simulink model "product_b1"  (R2021a)
settings: Solver=VariableStepAuto  StartTime=0.0  StopTime=10  FixedStep=0.001  RelTol=1e-3
InitFcn:
  | PreFunction.BusData
values from neighbouring files (symbols this model uses):
  N = 10    [TrajectoryGenerator.m]
undefined symbols (not defined in the file or in its folder): X, Y, Z
libraries: nesl_utility x29, sm_lib x24
settings Model: Creator=hanli  LastModifiedBy=hanli

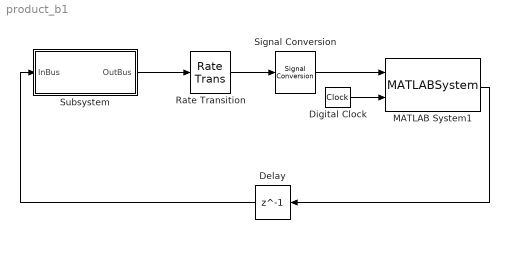
== system product_b1 ==
  Delay : Delay  DelayLength=1  InitialCondition=0  SampleTime=0.001
  Digital Clock : DigitalClock
  MATLAB System1 : MATLABSystem  System=EmptyController  SimulateUsing=Code generation
      mask Type: EmptyController
      mask Display:
      | disp('EmptyController');
      | port_label('input',1,'u');
      | port_label('input',2,'t');
      | port_label('output',1,'y');
  Rate Transition : RateTransition  OutPortSampleTime=0.001
  Signal Conversion : SignalConversion  ConversionOutput=Nonvirtual bus  OutDataTypeStr=Bus: AmberB1OutBus  OverrideOpt=off
  Subsystem : Subsystem
  wires:
  Subsystem/1(OutBus) -> Rate Transition/1
  Rate Transition/1 -> Signal Conversion/1
  Signal Conversion/1 -> MATLAB System1/1
  Delay/1 -> Subsystem/1(InBus)
  MATLAB System1/1 -> Delay/1
  Digital Clock/1 -> MATLAB System1/2

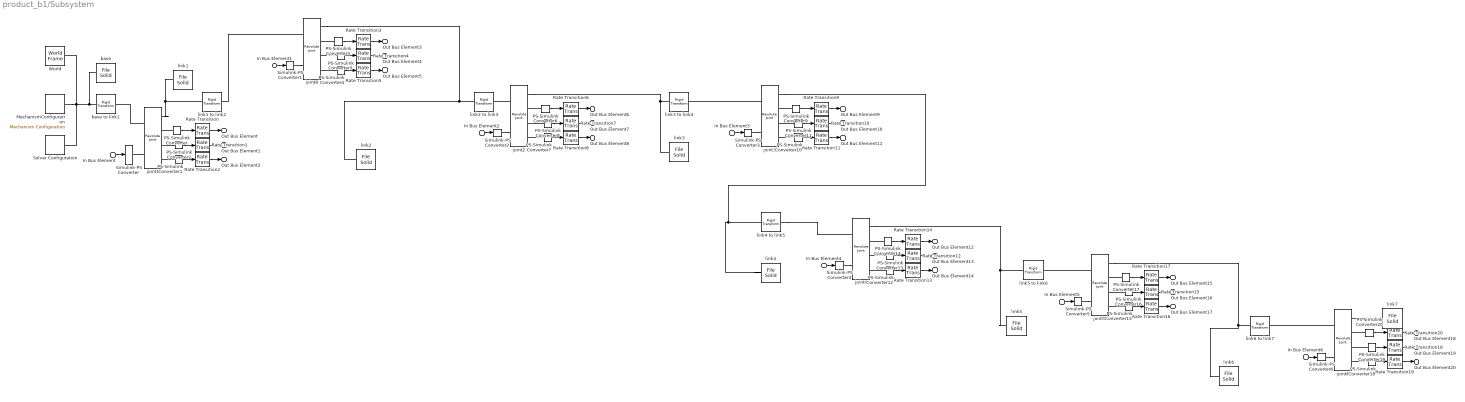
== system product_b1/Subsystem ==
  In Bus Element : Inport  PortName=InBus  Element=position_1
  In Bus Element1 : Inport  PortName=InBus  Element=position_2
  In Bus Element2 : Inport  PortName=InBus  Element=position_3
  In Bus Element3 : Inport  PortName=InBus  Element=position_4
  In Bus Element4 : Inport  PortName=InBus  Element=position_5
  In Bus Element5 : Inport  PortName=InBus  Element=position_6
  In Bus Element6 : Inport  PortName=InBus  Element=position_7
  MechanismConfiguration : sm_lib/Utilities/Mechanism Configuration  UniformGravity=Constant  GravityVector=[0 0 -9.80665]  GravityVectorUnits=m/s^2  GravityUnits=m/s^2  LinearizationDelta=0.001  JointModeTransitionNonlinearIterations=2
  PS-Simulink Converter{,1..20} (21 alike) : nesl_utility/PS-Simulink Converter  PhysicalDomain=network_engine_domain  SubClassName=ps_output  LeftPortType=input  RightPortType=output  PseudoPeriodic=off  Frequencies=[]  Unit=inherit  AffineConversion=off
      settings: SourceProductBaseCode=PW,SS
  Rate Transition{,1..20} (21 alike) : RateTransition  OutPortSampleTime=0.001
  Simulink-PS Converter{,1..6} (7 alike) : nesl_utility/Simulink-PS Converter  PhysicalDomain=network_engine_domain  SubClassName=ps_input  LeftPortType=input  RightPortType=output  PseudoPeriodic=off  Frequencies=[]  NoiseDistribution=none  NoiseParameters=[]  Unit=rad  AffineConversion=off  FilteringAndDerivatives=filter  SimscapeFilterOrder=2  InputFilterTimeConstant=0.001  UdotUserProvided=0
      settings: SourceProductBaseCode=PW,SS
  Solver Configuration : nesl_utility/Solver Configuration  PhysicalDomain=network_engine_domain  SubClassName=solver  LeftPortType=input  RightPortType=generic  Tones=[]  Harmonics=[]  SimulateNoise=off  Profile=off  UseLocalSampling=off  EnableSwitchedLinearOptims=on  FrequencyDomain=off  UseCCode=off  RelTol=0.001  AbsTol=1e-06  MinStep=1e-09  ToWorkspace=off  RevertToSquareIcSolve=off  NumHomotopyIterations=100  PhasorMode=off  PhasorModeNumHarmonics=1  DoDC=off  ResidualTolerance=1e-09  UseLocalSolver=off  LocalSolverChoice=NE_BACKWARD_EULER_ADVANCER  LocalSolverSampleTime=0.001  DoFixedCost=off  MaxNonlinIter=3  MaxModeIter=2  ComputeImpulses=off  ImpulseIterations=2  LinearAlgebra=auto  EquationFormulation=NE_TIME_EF  DelaysMemoryBudget=1024  AutomaticFiltering=on  FilteringTimeConstant=0.001  PartitionStorageMethod=AS_NEEDED  PartitionMemoryBudget=1024  PartitionMethod=ROBUST
      settings: SourceProductBaseCode=PW,SS
  World : sm_lib/Frames and Transforms/World Frame
  base : sm_lib/Body Elements/File Solid  ExtGeomFileName=meshes/base_link.STL  UnitType=Custom  ExtGeomFileUnits=m  StepReaderType=HEX  ExportConvexHullGeometry=off  InertiaType=Custom  Mass=0.26734  MassUnits=kg  CenterOfMass=[6.237e-05, 0.00031998, 0.048235]  CenterOfMassUnits=m  MomentsOfInertia=[0.00029777, 0.00024467, 0.00035934]  MomentsOfInertiaUnits=kg*m^2  ProductsOfInertia=[2.2995e-07, -3.3641e-08, 5.8953e-08]  ProductsOfInertiaUnits=kg*m^2  BasedOnType=DensityFromFile  Density=1000  DensityUnits=kg/m^3  DoExposeReferenceFrame=on  SerializedFrames=<Frames/>  GraphicType=FromGeometry  MarkerShape=Sphere  MarkerSize=10  GraphicVisPropType=SimpleVisualProperties  GraphicDiffuseColor=[0.62745, 0.62745, 0.62745]  GraphicSpecularColor=[0.5 0.5 0.5 1.0]  GraphicAmbientColor=[0.15 0.15 0.15 1.0]  GraphicEmissiveColor=[0.0 0.0 0.0 1.0]  GraphicShininess=75  GraphicOpacity=1
  base to link1 : sm_lib/Frames and Transforms/Rigid Transform  TranslationMethod=Cartesian  TranslationStandardOffset=0  TranslationLengthUnit=m  TranslationStandardAxis=+Z  TranslationCartesianOffset=[0, 0, 0.082]  TranslationROffset=0  TranslationROffsetUnits=m  TranslationZOffset=0  TranslationZOffsetUnits=m  TranslationThetaOffset=0  TranslationThetaOffsetUnits=deg  RotationMethod=RotationSequence  RotationAngleUnits=deg  RotationStandardAxis=+Z  RotationAngle=0.0  RotationArbitraryAxis=[0 0 1]  FollAlignAxisA=+X  BaseAlignAxisA=+Y  FollAlignAxisB=+Y  BaseAlignAxisB=+Z  RotationSequenceAxes=BaseAxes  RotationSequence=XYZ  RotationSequenceAngles=[0, 0, 0]  RotationSequenceAnglesUnits=rad  RotationMatrix=[1 0 0; 0 1 0; 0 0 1]
  joint1 : sm_lib/Joints/Revolute Joint  JointMode=Normal  SenseConstraintForce=off  SenseConstraintForceX=off  SenseConstraintForceY=off  SenseConstraintForceZ=off  SenseConstraintTorque=off  SenseConstraintTorqueX=off  SenseConstraintTorqueY=off  SenseConstraintTorqueZ=off  SenseTotalForce=off  SenseTotalForceX=off  SenseTotalForceY=off  SenseTotalForceZ=off  SenseTotalTorque=off  SenseTotalTorqueX=off  SenseTotalTorqueY=off  SenseTotalTorqueZ=off  CompositeWrenchDir=FollowerOnBase  CompositeWrenchFrame=BaseFrame  EquilibriumPosition=0  EquilibriumPositionUnits=deg  SpringStiffness=0  SpringStiffnessUnits=N*m/deg  DampingCoefficient=0.1  DampingCoefficientUnits=m^2*kg/s/rad  TorqueActuationMode=ComputedTorque  MotionActuationMode=InputMotion  SensePosition=on  SenseVelocity=on  SenseAcceleration=off  SenseTorqueForce=on  SenseLowerLimitTorqueForce=off  SenseUpperLimitTorqueForce=off  LowerLimitSpecify=on  LowerLimitBound=-2.4435  LowerLimitBoundUnits=rad  LowerLimitStiffness=1e4  LowerLimitStiffnessUnits=N*m/deg  LowerLimitDamping=10  LowerLimitDampingUnits=N*m/(deg/s)  LowerLimitTransitionRegionWidth=0.1  LowerLimitTransitionRegionWidthUnits=deg  UpperLimitSpecify=on  UpperLimitBound=2.4435  UpperLimitBoundUnits=rad  UpperLimitStiffness=1e4  UpperLimitStiffnessUnits=N*m/deg  UpperLimitDamping=10  UpperLimitDampingUnits=N*m/(deg/s)  UpperLimitTransitionRegionWidth=0.1  UpperLimitTransitionRegionWidthUnits=deg  PositionTargetSpecify=off  PositionTargetPriority=High  PositionTargetValue=0  PositionTargetValueUnits=deg  VelocityTargetSpecify=off  VelocityTargetPriority=High  VelocityTargetValue=0  VelocityTargetValueUnits=deg/s
  joint{2..5} (4 alike) : sm_lib/Joints/Revolute Joint  JointMode=Normal  SenseConstraintForce=off  SenseConstraintForceX=off  SenseConstraintForceY=off  SenseConstraintForceZ=off  SenseConstraintTorque=off  SenseConstraintTorqueX=off  SenseConstraintTorqueY=off  SenseConstraintTorqueZ=off  SenseTotalForce=off  SenseTotalForceX=off  SenseTotalForceY=off  SenseTotalForceZ=off  SenseTotalTorque=off  SenseTotalTorqueX=off  SenseTotalTorqueY=off  SenseTotalTorqueZ=off  CompositeWrenchDir=FollowerOnBase  CompositeWrenchFrame=BaseFrame  EquilibriumPosition=0  EquilibriumPositionUnits=deg  SpringStiffness=0  SpringStiffnessUnits=N*m/deg  DampingCoefficient=0.1  DampingCoefficientUnits=m^2*kg/s/rad  TorqueActuationMode=ComputedTorque  MotionActuationMode=InputMotion  SensePosition=on  SenseVelocity=on  SenseAcceleration=off  SenseTorqueForce=on  SenseLowerLimitTorqueForce=off  SenseUpperLimitTorqueForce=off  LowerLimitSpecify=on  LowerLimitBound=-2.2863  LowerLimitBoundUnits=rad  LowerLimitStiffness=1e4  LowerLimitStiffnessUnits=N*m/deg  LowerLimitDamping=10  LowerLimitDampingUnits=N*m/(deg/s)  LowerLimitTransitionRegionWidth=0.1  LowerLimitTransitionRegionWidthUnits=deg  UpperLimitSpecify=on  UpperLimitBound=2.2863  UpperLimitBoundUnits=rad  UpperLimitStiffness=1e4  UpperLimitStiffnessUnits=N*m/deg  UpperLimitDamping=10  UpperLimitDampingUnits=N*m/(deg/s)  UpperLimitTransitionRegionWidth=0.1  UpperLimitTransitionRegionWidthUnits=deg  PositionTargetSpecify=off  PositionTargetPriority=High  PositionTargetValue=0  PositionTargetValueUnits=deg  VelocityTargetSpecify=off  VelocityTargetPriority=High  VelocityTargetValue=0  VelocityTargetValueUnits=deg/s
  joint6 : sm_lib/Joints/Revolute Joint  JointMode=Normal  SenseConstraintForce=off  SenseConstraintForceX=off  SenseConstraintForceY=off  SenseConstraintForceZ=off  SenseConstraintTorque=off  SenseConstraintTorqueX=off  SenseConstraintTorqueY=off  SenseConstraintTorqueZ=off  SenseTotalForce=off  SenseTotalForceX=off  SenseTotalForceY=off  SenseTotalForceZ=off  SenseTotalTorque=off  SenseTotalTorqueX=off  SenseTotalTorqueY=off  SenseTotalTorqueZ=off  CompositeWrenchDir=FollowerOnBase  CompositeWrenchFrame=BaseFrame  EquilibriumPosition=0  EquilibriumPositionUnits=deg  SpringStiffness=0  SpringStiffnessUnits=N*m/deg  DampingCoefficient=0.1  DampingCoefficientUnits=m^2*kg/s/rad  TorqueActuationMode=ComputedTorque  MotionActuationMode=InputMotion  SensePosition=on  SenseVelocity=on  SenseAcceleration=off  SenseTorqueForce=on  SenseLowerLimitTorqueForce=off  SenseUpperLimitTorqueForce=off  LowerLimitSpecify=off  LowerLimitBound=-2.2863  LowerLimitBoundUnits=rad  LowerLimitStiffness=1e4  LowerLimitStiffnessUnits=N*m/deg  LowerLimitDamping=10  LowerLimitDampingUnits=N*m/(deg/s)  LowerLimitTransitionRegionWidth=0.1  LowerLimitTransitionRegionWidthUnits=deg  UpperLimitSpecify=off  UpperLimitBound=2.2863  UpperLimitBoundUnits=rad  UpperLimitStiffness=1e4  UpperLimitStiffnessUnits=N*m/deg  UpperLimitDamping=10  UpperLimitDampingUnits=N*m/(deg/s)  UpperLimitTransitionRegionWidth=0.1  UpperLimitTransitionRegionWidthUnits=deg  PositionTargetSpecify=off  PositionTargetPriority=High  PositionTargetValue=0  PositionTargetValueUnits=deg  VelocityTargetSpecify=off  VelocityTargetPriority=High  VelocityTargetValue=0  VelocityTargetValueUnits=deg/s
  joint8 : sm_lib/Joints/Revolute Joint  JointMode=Normal  SenseConstraintForce=off  SenseConstraintForceX=off  SenseConstraintForceY=off  SenseConstraintForceZ=off  SenseConstraintTorque=off  SenseConstraintTorqueX=off  SenseConstraintTorqueY=off  SenseConstraintTorqueZ=off  SenseTotalForce=off  SenseTotalForceX=off  SenseTotalForceY=off  SenseTotalForceZ=off  SenseTotalTorque=off  SenseTotalTorqueX=off  SenseTotalTorqueY=off  SenseTotalTorqueZ=off  CompositeWrenchDir=FollowerOnBase  CompositeWrenchFrame=BaseFrame  EquilibriumPosition=0  EquilibriumPositionUnits=deg  SpringStiffness=0  SpringStiffnessUnits=N*m/deg  DampingCoefficient=0.1  DampingCoefficientUnits=m^2*kg/s/rad  TorqueActuationMode=ComputedTorque  MotionActuationMode=InputMotion  SensePosition=on  SenseVelocity=on  SenseAcceleration=off  SenseTorqueForce=on  SenseLowerLimitTorqueForce=off  SenseUpperLimitTorqueForce=off  LowerLimitSpecify=on  LowerLimitBound=-2.3213  LowerLimitBoundUnits=rad  LowerLimitStiffness=1e4  LowerLimitStiffnessUnits=N*m/deg  LowerLimitDamping=10  LowerLimitDampingUnits=N*m/(deg/s)  LowerLimitTransitionRegionWidth=0.1  LowerLimitTransitionRegionWidthUnits=deg  UpperLimitSpecify=on  UpperLimitBound=2.3213  UpperLimitBoundUnits=rad  UpperLimitStiffness=1e4  UpperLimitStiffnessUnits=N*m/deg  UpperLimitDamping=10  UpperLimitDampingUnits=N*m/(deg/s)  UpperLimitTransitionRegionWidth=0.1  UpperLimitTransitionRegionWidthUnits=deg  PositionTargetSpecify=off  PositionTargetPriority=High  PositionTargetValue=0  PositionTargetValueUnits=deg  VelocityTargetSpecify=off  VelocityTargetPriority=High  VelocityTargetValue=0  VelocityTargetValueUnits=deg/s
  link1 : sm_lib/Body Elements/File Solid  ExtGeomFileName=meshes/link1.STL  UnitType=Custom  ExtGeomFileUnits=m  StepReaderType=HEX  ExportConvexHullGeometry=off  InertiaType=Custom  Mass=0.2539  MassUnits=kg  CenterOfMass=[-7.1956e-05, -0.0006525, 0.065648]  CenterOfMassUnits=m  MomentsOfInertia=[0.00013206, 0.00021227, 0.00013113]  MomentsOfInertiaUnits=kg*m^2  ProductsOfInertia=[-7.2775e-06, 5.8071e-08, -1.112e-07]  ProductsOfInertiaUnits=kg*m^2  BasedOnType=DensityFromFile  Density=1000  DensityUnits=kg/m^3  DoExposeReferenceFrame=on  SerializedFrames=<Frames/>  GraphicType=FromGeometry  MarkerShape=Sphere  MarkerSize=10  GraphicVisPropType=SimpleVisualProperties  GraphicDiffuseColor=[0.83922, 0.44706, 0.38431]  GraphicSpecularColor=[0.5 0.5 0.5 1.0]  GraphicAmbientColor=[0.15 0.15 0.15 1.0]  GraphicEmissiveColor=[0.0 0.0 0.0 1.0]  GraphicShininess=75  GraphicOpacity=1
  link1 to link2 : sm_lib/Frames and Transforms/Rigid Transform  TranslationMethod=Cartesian  TranslationStandardOffset=0  TranslationLengthUnit=m  TranslationStandardAxis=+Z  TranslationCartesianOffset=[0, 0.025, 0.08649999999999999]  TranslationROffset=0  TranslationROffsetUnits=m  TranslationZOffset=0  TranslationZOffsetUnits=m  TranslationThetaOffset=0  TranslationThetaOffsetUnits=deg  RotationMethod=RotationSequence  RotationAngleUnits=deg  RotationStandardAxis=+Z  RotationAngle=0.0  RotationArbitraryAxis=[0 0 1]  FollAlignAxisA=+X  BaseAlignAxisA=+Y  FollAlignAxisB=+Y  BaseAlignAxisB=+Z  RotationSequenceAxes=BaseAxes  RotationSequence=XYZ  RotationSequenceAngles=[1.5708, 0, 3.1416]  RotationSequenceAnglesUnits=rad  RotationMatrix=[1 0 0; 0 1 0; 0 0 1]
  link2 : sm_lib/Body Elements/File Solid  ExtGeomFileName=meshes/link2.STL  UnitType=Custom  ExtGeomFileUnits=m  StepReaderType=HEX  ExportConvexHullGeometry=off  InertiaType=Custom  Mass=0.26004  MassUnits=kg  CenterOfMass=[5.7141e-05, 0.080805, -0.0071326]  CenterOfMassUnits=m  MomentsOfInertia=[0.00027467, 0.00015654, 0.00029313]  MomentsOfInertiaUnits=kg*m^2  ProductsOfInertia=[-3.0164e-06, 9.7156e-08, 1.0052e-07]  ProductsOfInertiaUnits=kg*m^2  BasedOnType=DensityFromFile  Density=1000  DensityUnits=kg/m^3  DoExposeReferenceFrame=on  SerializedFrames=<Frames/>  GraphicType=FromGeometry  MarkerShape=Sphere  MarkerSize=10  GraphicVisPropType=SimpleVisualProperties  GraphicDiffuseColor=[0.66667, 0.66667, 0.66667]  GraphicSpecularColor=[0.5 0.5 0.5 1.0]  GraphicAmbientColor=[0.15 0.15 0.15 1.0]  GraphicEmissiveColor=[0.0 0.0 0.0 1.0]  GraphicShininess=75  GraphicOpacity=1
  link2 to link3 : sm_lib/Frames and Transforms/Rigid Transform  TranslationMethod=Cartesian  TranslationStandardOffset=0  TranslationLengthUnit=m  TranslationStandardAxis=+Z  TranslationCartesianOffset=[0, 0.1364, -0.025]  TranslationROffset=0  TranslationROffsetUnits=m  TranslationZOffset=0  TranslationZOffsetUnits=m  TranslationThetaOffset=0  TranslationThetaOffsetUnits=deg  RotationMethod=RotationSequence  RotationAngleUnits=deg  RotationStandardAxis=+Z  RotationAngle=0.0  RotationArbitraryAxis=[0 0 1]  FollAlignAxisA=+X  BaseAlignAxisA=+Y  FollAlignAxisB=+Y  BaseAlignAxisB=+Z  RotationSequenceAxes=BaseAxes  RotationSequence=XYZ  RotationSequenceAngles=[1.5708, 0, 3.1416]  RotationSequenceAnglesUnits=rad  RotationMatrix=[1 0 0; 0 1 0; 0 0 1]
  link3 : sm_lib/Body Elements/File Solid  ExtGeomFileName=meshes/link3.STL  UnitType=Custom  ExtGeomFileUnits=m  StepReaderType=HEX  ExportConvexHullGeometry=off  InertiaType=Custom  Mass=0.19745  MassUnits=kg  CenterOfMass=[7.536e-05, 0.00081876, 0.06766999999999999]  CenterOfMassUnits=m  MomentsOfInertia=[8.8302e-05, 0.00014017, 8.488e-05]  MomentsOfInertiaUnits=kg*m^2  ProductsOfInertia=[5.8084e-06, -9.7553e-08, -1.0051e-07]  ProductsOfInertiaUnits=kg*m^2  BasedOnType=DensityFromFile  Density=1000  DensityUnits=kg/m^3  DoExposeReferenceFrame=on  SerializedFrames=<Frames/>  GraphicType=FromGeometry  MarkerShape=Sphere  MarkerSize=10  GraphicVisPropType=SimpleVisualProperties  GraphicDiffuseColor=[0.83922, 0.44706, 0.38431]  GraphicSpecularColor=[0.5 0.5 0.5 1.0]  GraphicAmbientColor=[0.15 0.15 0.15 1.0]  GraphicEmissiveColor=[0.0 0.0 0.0 1.0]  GraphicShininess=75  GraphicOpacity=1
  link3 to link4 : sm_lib/Frames and Transforms/Rigid Transform  TranslationMethod=Cartesian  TranslationStandardOffset=0  TranslationLengthUnit=m  TranslationStandardAxis=+Z  TranslationCartesianOffset=[0, -0.025, 0.08110000000000001]  TranslationROffset=0  TranslationROffsetUnits=m  TranslationZOffset=0  TranslationZOffsetUnits=m  TranslationThetaOffset=0  TranslationThetaOffsetUnits=deg  RotationMethod=RotationSequence  RotationAngleUnits=deg  RotationStandardAxis=+Z  RotationAngle=0.0  RotationArbitraryAxis=[0 0 1]  FollAlignAxisA=+X  BaseAlignAxisA=+Y  FollAlignAxisB=+Y  BaseAlignAxisB=+Z  RotationSequenceAxes=BaseAxes  RotationSequence=XYZ  RotationSequenceAngles=[1.5708, 0, 0]  RotationSequenceAnglesUnits=rad  RotationMatrix=[1 0 0; 0 1 0; 0 0 1]
  link4 : sm_lib/Body Elements/File Solid  ExtGeomFileName=meshes/link4.STL  UnitType=Custom  ExtGeomFileUnits=m  StepReaderType=HEX  ExportConvexHullGeometry=off  InertiaType=Custom  Mass=0.2255  MassUnits=kg  CenterOfMass=[5.5658e-05, 0.075812, -0.010096]  CenterOfMassUnits=m  MomentsOfInertia=[0.00018432, 0.00014008, 0.00019346]  MomentsOfInertiaUnits=kg*m^2  ProductsOfInertia=[5.464e-09, 9.3583e-08, 9.341e-08]  ProductsOfInertiaUnits=kg*m^2  BasedOnType=DensityFromFile  Density=1000  DensityUnits=kg/m^3  DoExposeReferenceFrame=on  SerializedFrames=<Frames/>  GraphicType=FromGeometry  MarkerShape=Sphere  MarkerSize=10  GraphicVisPropType=SimpleVisualProperties  GraphicDiffuseColor=[0.66667, 0.66667, 0.66667]  GraphicSpecularColor=[0.5 0.5 0.5 1.0]  GraphicAmbientColor=[0.15 0.15 0.15 1.0]  GraphicEmissiveColor=[0.0 0.0 0.0 1.0]  GraphicShininess=75  GraphicOpacity=1
  link4 to link5 : sm_lib/Frames and Transforms/Rigid Transform  TranslationMethod=Cartesian  TranslationStandardOffset=0  TranslationLengthUnit=m  TranslationStandardAxis=+Z  TranslationCartesianOffset=[0, 0.121, -0.025]  TranslationROffset=0  TranslationROffsetUnits=m  TranslationZOffset=0  TranslationZOffsetUnits=m  TranslationThetaOffset=0  TranslationThetaOffsetUnits=deg  RotationMethod=RotationSequence  RotationAngleUnits=deg  RotationStandardAxis=+Z  RotationAngle=0.0  RotationArbitraryAxis=[0 0 1]  FollAlignAxisA=+X  BaseAlignAxisA=+Y  FollAlignAxisB=+Y  BaseAlignAxisB=+Z  RotationSequenceAxes=BaseAxes  RotationSequence=XYZ  RotationSequenceAngles=[-1.5708, 0, 0]  RotationSequenceAnglesUnits=rad  RotationMatrix=[1 0 0; 0 1 0; 0 0 1]
  link5 : sm_lib/Body Elements/File Solid  ExtGeomFileName=meshes/link5.STL  UnitType=Custom  ExtGeomFileUnits=m  StepReaderType=HEX  ExportConvexHullGeometry=off  InertiaType=Custom  Mass=0.188342091601826  MassUnits=kg  CenterOfMass=[-6.47608224975801e-05, -0.000135644729966451, 0.0681146474008698]  CenterOfMassUnits=m  MomentsOfInertia=[8.572084994320241e-05, 0.000135395618146542, 8.20376711496822e-05]  MomentsOfInertiaUnits=kg*m^2  ProductsOfInertia=[-5.79908404802222e-06, 9.3610025889588e-08, -9.362853198210679e-08]  ProductsOfInertiaUnits=kg*m^2  BasedOnType=DensityFromFile  Density=1000  DensityUnits=kg/m^3  DoExposeReferenceFrame=on  SerializedFrames=<Frames/>  GraphicType=FromGeometry  MarkerShape=Sphere  MarkerSize=10  GraphicVisPropType=SimpleVisualProperties  GraphicDiffuseColor=[0.83921568627451, 0.447058823529412, 0.384313725490196]  GraphicSpecularColor=[0.5 0.5 0.5 1.0]  GraphicAmbientColor=[0.15 0.15 0.15 1.0]  GraphicEmissiveColor=[0.0 0.0 0.0 1.0]  GraphicShininess=75  GraphicOpacity=1
  link5 to link6 : sm_lib/Frames and Transforms/Rigid Transform  TranslationMethod=Cartesian  TranslationStandardOffset=0  TranslationLengthUnit=m  TranslationStandardAxis=+Z  TranslationCartesianOffset=[0, 0.025, 0.08110000000000001]  TranslationROffset=0  TranslationROffsetUnits=m  TranslationZOffset=0  TranslationZOffsetUnits=m  TranslationThetaOffset=0  TranslationThetaOffsetUnits=deg  RotationMethod=RotationSequence  RotationAngleUnits=deg  RotationStandardAxis=+Z  RotationAngle=0.0  RotationArbitraryAxis=[0 0 1]  FollAlignAxisA=+X  BaseAlignAxisA=+Y  FollAlignAxisB=+Y  BaseAlignAxisB=+Z  RotationSequenceAxes=BaseAxes  RotationSequence=XYZ  RotationSequenceAngles=[-1.5708, 0, 0]  RotationSequenceAnglesUnits=rad  RotationMatrix=[1 0 0; 0 1 0; 0 0 1]
  link6 : sm_lib/Body Elements/File Solid  ExtGeomFileName=meshes/link6.STL  UnitType=Custom  ExtGeomFileUnits=m  StepReaderType=HEX  ExportConvexHullGeometry=off  InertiaType=Custom  Mass=0.228014101529845  MassUnits=kg  CenterOfMass=[-5.3512302833054e-05, -0.0764997090438678, -0.0106346714964407]  CenterOfMassUnits=m  MomentsOfInertia=[0.000184226138693011, 0.000140231791267273, 0.000193377959750286]  MomentsOfInertiaUnits=kg*m^2  ProductsOfInertia=[-9.861040295655519e-09, -9.35833296390346e-08, 9.34105969132088e-08]  ProductsOfInertiaUnits=kg*m^2  BasedOnType=DensityFromFile  Density=1000  DensityUnits=kg/m^3  DoExposeReferenceFrame=on  SerializedFrames=<Frames/>  GraphicType=FromGeometry  MarkerShape=Sphere  MarkerSize=10  GraphicVisPropType=SimpleVisualProperties  GraphicDiffuseColor=[0.666666666666667, 0.666666666666667, 0.666666666666667]  GraphicSpecularColor=[0.5 0.5 0.5 1.0]  GraphicAmbientColor=[0.15 0.15 0.15 1.0]  GraphicEmissiveColor=[0.0 0.0 0.0 1.0]  GraphicShininess=75  GraphicOpacity=1
  link6 to link7 : sm_lib/Frames and Transforms/Rigid Transform  TranslationMethod=Cartesian  TranslationStandardOffset=0  TranslationLengthUnit=m  TranslationStandardAxis=+Z  TranslationCartesianOffset=[0, -0.121, -0.025]  TranslationROffset=0  TranslationROffsetUnits=m  TranslationZOffset=0  TranslationZOffsetUnits=m  TranslationThetaOffset=0  TranslationThetaOffsetUnits=deg  RotationMethod=RotationSequence  RotationAngleUnits=deg  RotationStandardAxis=+Z  RotationAngle=0.0  RotationArbitraryAxis=[0 0 1]  FollAlignAxisA=+X  BaseAlignAxisA=+Y  FollAlignAxisB=+Y  BaseAlignAxisB=+Z  RotationSequenceAxes=BaseAxes  RotationSequence=XYZ  RotationSequenceAngles=[1.5708, 0, 0]  RotationSequenceAnglesUnits=rad  RotationMatrix=[1 0 0; 0 1 0; 0 0 1]
  link7 : sm_lib/Body Elements/File Solid  ExtGeomFileName=meshes/link7.STL  UnitType=Custom  ExtGeomFileUnits=m  StepReaderType=HEX  ExportConvexHullGeometry=off  InertiaType=Custom  Mass=0.030725  MassUnits=kg  CenterOfMass=[-1.5306e-10, 3.6809e-05, 0.020162]  CenterOfMassUnits=m  MomentsOfInertia=[9.1931e-06, 9.217e-06, 8.090299999999999e-06]  MomentsOfInertiaUnits=kg*m^2  ProductsOfInertia=[1.7076e-08, -7.0127e-14, 1.8624e-13]  ProductsOfInertiaUnits=kg*m^2  BasedOnType=DensityFromFile  Density=1000  DensityUnits=kg/m^3  DoExposeReferenceFrame=on  SerializedFrames=<Frames/>  GraphicType=FromGeometry  MarkerShape=Sphere  MarkerSize=10  GraphicVisPropType=SimpleVisualProperties  GraphicDiffuseColor=[0.94902, 0.75686, 0.17647]  GraphicSpecularColor=[0.5 0.5 0.5 1.0]  GraphicAmbientColor=[0.15 0.15 0.15 1.0]  GraphicEmissiveColor=[0.0 0.0 0.0 1.0]  GraphicShininess=75  GraphicOpacity=1
  Out Bus Element : Outport  PortName=OutBus  Element=joint_1.position
  Out Bus Element1 : Outport  PortName=OutBus  Element=joint_1.velocity
  Out Bus Element2 : Outport  PortName=OutBus  Element=joint_1.torque
  Out Bus Element3 : Outport  PortName=OutBus  Element=joint_2.position
  Out Bus Element4 : Outport  PortName=OutBus  Element=joint_2.velocity
  Out Bus Element5 : Outport  PortName=OutBus  Element=joint_2.torque
  Out Bus Element6 : Outport  PortName=OutBus  Element=joint_3.position
  Out Bus Element7 : Outport  PortName=OutBus  Element=joint_3.velocity
  Out Bus Element8 : Outport  PortName=OutBus  Element=joint_3.torque
  Out Bus Element9 : Outport  PortName=OutBus  Element=joint_4.position
  Out Bus Element10 : Outport  PortName=OutBus  Element=joint_4.velocity
  Out Bus Element11 : Outport  PortName=OutBus  Element=joint_4.torque
  Out Bus Element12 : Outport  PortName=OutBus  Element=joint_5.position
  Out Bus Element13 : Outport  PortName=OutBus  Element=joint_5.velocity
  Out Bus Element14 : Outport  PortName=OutBus  Element=joint_5.torque
  Out Bus Element15 : Outport  PortName=OutBus  Element=joint_6.position
  Out Bus Element16 : Outport  PortName=OutBus  Element=joint_6.velocity
  Out Bus Element17 : Outport  PortName=OutBus  Element=joint_6.torque
  Out Bus Element18 : Outport  PortName=OutBus  Element=joint_7.position
  Out Bus Element19 : Outport  PortName=OutBus  Element=joint_7.velocity
  Out Bus Element20 : Outport  PortName=OutBus  Element=joint_7.torque
  wires:
  In Bus Element/1 -> Simulink-PS Converter/1
  PS-Simulink Converter/1 -> Rate Transition/1
  PS-Simulink Converter2/1 -> Rate Transition1/1
  PS-Simulink Converter1/1 -> Rate Transition2/1
  Rate Transition2/1 -> Out Bus Element2/1
  Rate Transition1/1 -> Out Bus Element1/1
  Rate Transition/1 -> Out Bus Element/1
  Rate Transition3/1 -> Out Bus Element3/1
  Rate Transition4/1 -> Out Bus Element4/1
  PS-Simulink Converter5/1 -> Rate Transition4/1
  Rate Transition5/1 -> Out Bus Element5/1
  In Bus Element1/1 -> Simulink-PS Converter1/1
  PS-Simulink Converter3/1 -> Rate Transition3/1
  PS-Simulink Converter4/1 -> Rate Transition5/1
  PS-Simulink Converter7/1 -> Rate Transition8/1
  PS-Simulink Converter6/1 -> Rate Transition6/1
  In Bus Element2/1 -> Simulink-PS Converter2/1
  Rate Transition8/1 -> Out Bus Element8/1
  PS-Simulink Converter8/1 -> Rate Transition7/1
  Rate Transition7/1 -> Out Bus Element7/1
  Rate Transition6/1 -> Out Bus Element6/1
  PS-Simulink Converter10/1 -> Rate Transition11/1
  PS-Simulink Converter9/1 -> Rate Transition9/1
  In Bus Element3/1 -> Simulink-PS Converter3/1
  Rate Transition11/1 -> Out Bus Element11/1
  Rate Transition10/1 -> Out Bus Element10/1
  PS-Simulink Converter11/1 -> Rate Transition10/1
  Rate Transition9/1 -> Out Bus Element9/1
  Rate Transition12/1 -> Out Bus Element13/1
  Rate Transition13/1 -> Out Bus Element14/1
  In Bus Element4/1 -> Simulink-PS Converter4/1
  PS-Simulink Converter13/1 -> Rate Transition12/1
  PS-Simulink Converter12/1 -> Rate Transition13/1
  Rate Transition14/1 -> Out Bus Element12/1
  PS-Simulink Converter14/1 -> Rate Transition14/1
  PS-Simulink Converter15/1 -> Rate Transition16/1
  Rate Transition17/1 -> Out Bus Element15/1
  Rate Transition15/1 -> Out Bus Element16/1
  In Bus Element5/1 -> Simulink-PS Converter5/1
  Rate Transition16/1 -> Out Bus Element17/1
  PS-Simulink Converter17/1 -> Rate Transition17/1
  PS-Simulink Converter16/1 -> Rate Transition15/1
  PS-Simulink Converter18/1 -> Rate Transition19/1
  Rate Transition20/1 -> Out Bus Element18/1
  Rate Transition18/1 -> Out Bus Element19/1
  In Bus Element6/1 -> Simulink-PS Converter6/1
  Rate Transition19/1 -> Out Bus Element20/1
  PS-Simulink Converter20/1 -> Rate Transition20/1
  PS-Simulink Converter19/1 -> Rate Transition18/1
  connections:
  MechanismConfiguration/RConn1 -- Solver Configuration/RConn1 -- World/RConn1 -- base/RConn1 -- base to link1/LConn1
  joint1/LConn1 -- base to link1/RConn1
  link3/RConn1 -- joint2/RConn1 -- link3 to link4/LConn1
  link4/RConn1 -- joint3/RConn1 -- link4 to link5/LConn1
  link2/RConn1 -- joint8/RConn1 -- link2 to link3/LConn1
  link6 to link7/LConn1 -- link6/RConn1 -- joint5/RConn1
  link5/RConn1 -- joint4/RConn1 -- link5 to link6/LConn1
  joint1/RConn1 -- link1/RConn1 -- link1 to link2/LConn1
  Simulink-PS Converter/RConn1 -- joint1/LConn2
  PS-Simulink Converter/LConn1 -- joint1/RConn2
  PS-Simulink Converter2/LConn1 -- joint1/RConn3
  PS-Simulink Converter1/LConn1 -- joint1/RConn4
  Simulink-PS Converter1/RConn1 -- joint8/LConn2
  PS-Simulink Converter5/LConn1 -- joint8/RConn3
  PS-Simulink Converter4/LConn1 -- joint8/RConn4
  PS-Simulink Converter3/LConn1 -- joint8/RConn2
  link1 to link2/RConn1 -- joint8/LConn1
  PS-Simulink Converter6/LConn1 -- joint2/RConn2
  PS-Simulink Converter7/LConn1 -- joint2/RConn4
  PS-Simulink Converter8/LConn1 -- joint2/RConn3
  Simulink-PS Converter2/RConn1 -- joint2/LConn2
  joint2/LConn1 -- link2 to link3/RConn1
  PS-Simulink Converter10/LConn1 -- joint3/RConn4
  PS-Simulink Converter9/LConn1 -- joint3/RConn2
  PS-Simulink Converter11/LConn1 -- joint3/RConn3
  Simulink-PS Converter3/RConn1 -- joint3/LConn2
  joint3/LConn1 -- link3 to link4/RConn1
  PS-Simulink Converter12/LConn1 -- joint4/RConn4
  PS-Simulink Converter13/LConn1 -- joint4/RConn3
  Simulink-PS Converter4/RConn1 -- joint4/LConn2
  PS-Simulink Converter14/LConn1 -- joint4/RConn2
  link4 to link5/RConn1 -- joint4/LConn1
  PS-Simulink Converter16/LConn1 -- joint5/RConn3
  Simulink-PS Converter5/RConn1 -- joint5/LConn2
  PS-Simulink Converter15/LConn1 -- joint5/RConn4
  PS-Simulink Converter17/LConn1 -- joint5/RConn2
  joint5/LConn1 -- link5 to link6/RConn1
  PS-Simulink Converter19/LConn1 -- joint6/RConn3
  Simulink-PS Converter6/RConn1 -- joint6/LConn2
  PS-Simulink Converter18/LConn1 -- joint6/RConn4
  PS-Simulink Converter20/LConn1 -- joint6/RConn2
  link7/RConn1 -- joint6/RConn1
  joint6/LConn1 -- link6 to link7/RConn1
